simulink model "predador_presa"  (R2015a)
settings: Solver=ode45  StartTime=0.0  StopTime=tsim  RelTol=1e-3
values from neighbouring files (symbols this model uses):
  alpha1 = 1.4    [erro.m]    (also in lab1.m)
  alpha2 = alpha2_aux(i)    [Untitled.m]    (also in erro.m = parametros(2); lab1.m = optimo(2))
  delta1 = 3.1    [erro.m]    (also in lab1.m)
  delta2 = -1.5    [erro.m]    (also in lab1.m)
  N10 = 4    [erro.m]    (also in lab1.m)
  N20 = N20_aux(j)    [Untitled.m]    (also in erro.m = parametros(1); lab1.m = optimo(1))
settings Model: Creator=Alunos  LastModifiedBy=Diogo

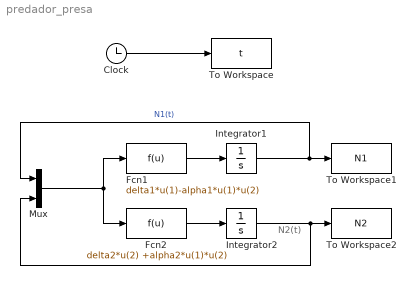
== system predador_presa ==
  note: N2(t)
  Clock : Clock
  Fcn1 : Fcn  Expr=delta1*u(1)-alpha1*u(1)*u(2)
  Fcn2 : Fcn  Expr=delta2*u(2) +alpha2*u(1)*u(2)
  Integrator1 : Integrator  InitialCondition=N10
  Integrator2 : Integrator  InitialCondition=N20
  Mux : Mux  Inputs=2
  To Workspace : ToWorkspace  VariableName=t  SampleTime=-1
  To Workspace1 : ToWorkspace  VariableName=N1  SampleTime=-1
  To Workspace2 : ToWorkspace  VariableName=N2  SampleTime=-1
  wires:
  Clock/1 -> To Workspace/1
  Integrator1/1 -> Mux/1, To Workspace1/1  "N1(t)"
  Fcn2/1 -> Integrator2/1
  Fcn1/1 -> Integrator1/1
  Mux/1 -> Fcn2/1, Fcn1/1
  Integrator2/1 -> Mux/2, To Workspace2/1
